simulink model "Regulation_task_cartesian_and_posture"  (R2025b)
settings: Solver=VariableStepAuto  StartTime=0.0  StopTime=10.0  RelTol=1e-3
values from neighbouring files (symbols this model uses):
  k1 = 2 * zeta * g    (= 9.6)    [test1.m]
  k2 = g^2    (= 64)    [test1.m]
  k3 = k1    (= 9.6)    [test1.m]
undefined symbols (not defined in the file or in its folder): shift_time
settings Model: Creator=david  LastModifiedBy=david

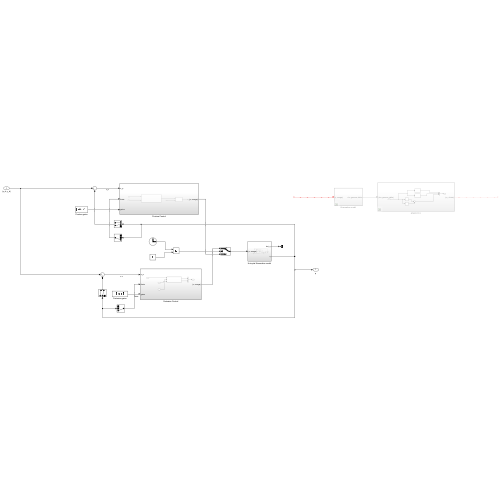
[thumbnail: Simulink's stored preview of the top-level diagram]
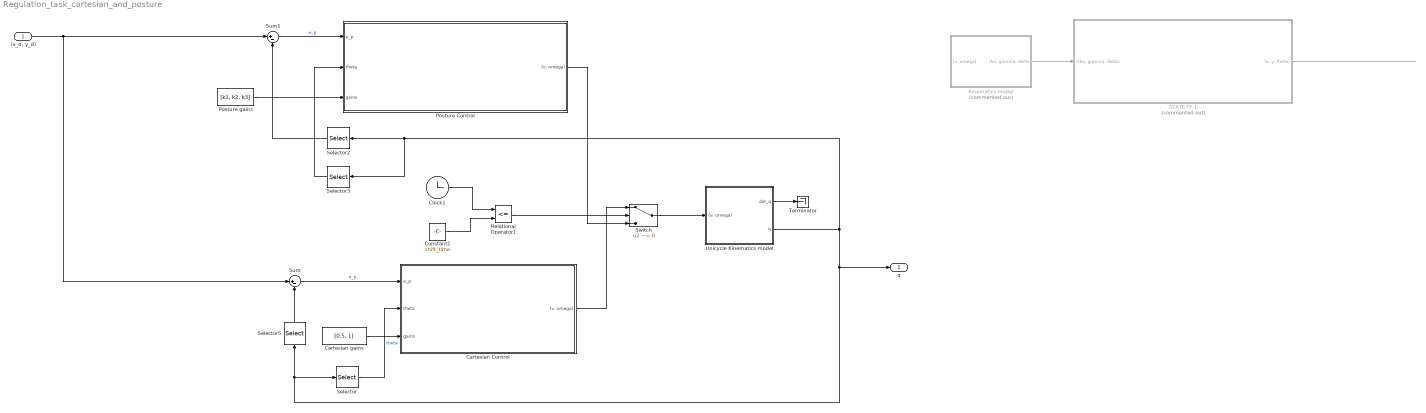
== system Regulation_task_cartesian_and_posture ==
  "(x_d, y_d)" : Inport
  Cartesian Control : Subsystem
  Cartesian gains : Constant  Value=[0.5, 1]
  Clock1 : Clock
  Constant1 : Constant  Value=shift_time
  Kinematics model : Subsystem  Commented=on
  Posture Control : Subsystem
  Posture gains : Constant  Value=[k1, k2, k3]
  Relational Operator1 : RelationalOperator  Operator=<=  OutDataTypeStr=boolean  RndMeth=Simplest  InputSameDT=off
  STATE TF-1 : Subsystem  Commented=on
  Selector : Selector  InputPortWidth=3  IndexOptions=Index vector (dialog)  Indices=[3]  OutputSizes=1
  Selector2 : Selector  InputPortWidth=3  IndexOptions=Index vector (dialog)  Indices=[1 2]  OutputSizes=1
  Selector3 : Selector  InputPortWidth=3  IndexOptions=Index vector (dialog)  Indices=[3]  OutputSizes=1
  Selector5 : Selector  InputPortWidth=3  IndexOptions=Index vector (dialog)  Indices=[1 2]  OutputSizes=1
  Sum : Sum  Inputs=|+-
  Sum1 : Sum  Inputs=|+-
  Switch : Switch  Criteria=u2 ~= 0  Threshold=0.1  SaturateOnIntegerOverflow=off  InputSameDT=off
  Terminator : Terminator
  Unicycle Kinematics model : Subsystem
  q : Outport
  wires:
  Sum/1 -> Cartesian Control/1(e_p)  "e_p"
  Selector/1 -> Cartesian Control/2(theta)  "theta"
  Unicycle Kinematics model/2(q) -> Selector3/1, Selector2/1, q/1, Selector5/1, Selector/1
  Cartesian gains/1 -> Cartesian Control/3(gains)
  STATE TF-1/1("(x, y, theta)") -> ?
  Kinematics model/1("rho, gamma, delta") -> STATE TF-1/1("(rho, gamma, delta)")
  Selector2/1 -> Sum1/2
  Sum1/1 -> Posture Control/1(e_p)  "e_p"
  Selector3/1 -> Posture Control/2(theta)
  Unicycle Kinematics model/1(dot_q) -> Terminator/1
  Cartesian Control/1("(v, omega)") -> Switch/1
  ? -> Kinematics model/1("(v, omega)")
  Switch/1 -> Unicycle Kinematics model/1("(v, omega)")
  Posture Control/1("(v, omega)") -> Switch/3
  "(x_d, y_d)"/1 -> Sum/1, Sum1/1
  Selector5/1 -> Sum/2
  Posture gains/1 -> Posture Control/3(gains)
  Relational Operator1/1 -> Switch/2
  Clock1/1 -> Relational Operator1/1
  Constant1/1 -> Relational Operator1/2

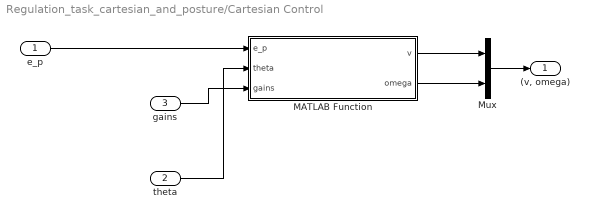
== system Regulation_task_cartesian_and_posture/Cartesian Control ==
  e_p : Inport
  theta : Inport  Port=2
  gains : Inport  Port=3
  MATLAB Function : MATLAB Function  TreatAsAtomicUnit=on
  Mux : Mux  Inputs=2
  "(v, omega)" : Outport
  wires:
  e_p/1 -> MATLAB Function/1(e_p)
  gains/1 -> MATLAB Function/3(gains)
  theta/1 -> MATLAB Function/2(theta)
  MATLAB Function/2(omega) -> Mux/2
  MATLAB Function/1(v) -> Mux/1
  Mux/1 -> "(v, omega)"/1

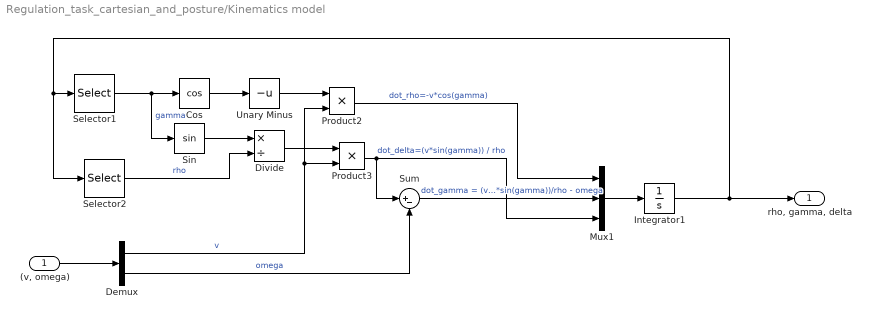
== system Regulation_task_cartesian_and_posture/Kinematics model ==
  "(v, omega)" : Inport
  Cos : Trigonometry  Operator=cos
  Demux : Demux  Outputs=2
  Divide : Product  Inputs=*/
  Integrator1 : Integrator
  Mux1 : Mux  Inputs=3
  Product2 : Product
  Product3 : Product
  Selector1 : Selector  InputPortWidth=3  IndexOptions=Index vector (dialog)  Indices=[2]  OutputSizes=1
  Selector2 : Selector  InputPortWidth=3  IndexOptions=Index vector (dialog)  Indices=[1]  OutputSizes=1
  Sin : Trigonometry
  Sum : Sum  Inputs=|+-
  Unary Minus : UnaryMinus
  "rho, gamma, delta" : Outport
  wires:
  Integrator1/1 -> "rho, gamma, delta"/1, Selector2/1, Selector1/1
  "(v, omega)"/1 -> Demux/1
  Mux1/1 -> Integrator1/1
  Selector1/1 -> Sin/1, Cos/1  "gamma"
  Cos/1 -> Unary Minus/1
  Unary Minus/1 -> Product2/1
  Demux/1 -> Product3/2, Product2/2  "v"
  Sin/1 -> Divide/1
  Selector2/1 -> Divide/2  "rho"
  Divide/1 -> Product3/1
  Product2/1 -> Mux1/1  "dot_rho=-v*cos(gamma)"
  Product3/1 -> Sum/1, Mux1/3  "dot_delta=(v*sin(gamma)) / rho"
  Sum/1 -> Mux1/2  "dot_gamma = (v*sin(gamma))/rho - omega"
  Demux/2 -> Sum/2  "omega"

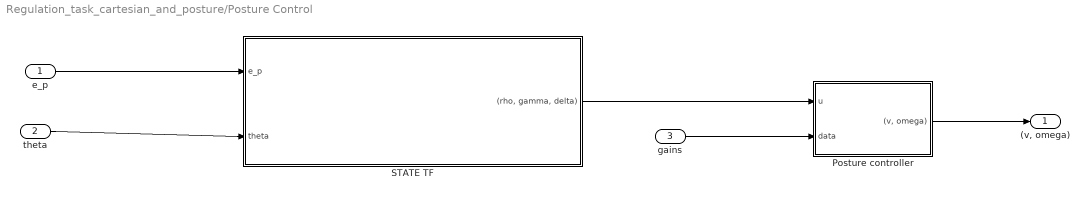
== system Regulation_task_cartesian_and_posture/Posture Control ==
  e_p : Inport
  theta : Inport  Port=2
  gains : Inport  Port=3
  Posture controller : Subsystem
  "STATE TF " : Subsystem
  "(v, omega)" : Outport
  wires:
  gains/1 -> Posture controller/2(data)
  theta/1 -> "STATE TF "/2(theta)
  "STATE TF "/1("(rho, gamma, delta)") -> Posture controller/1(u)
  Posture controller/1("(v, omega)") -> "(v, omega)"/1
  e_p/1 -> "STATE TF "/1(e_p)

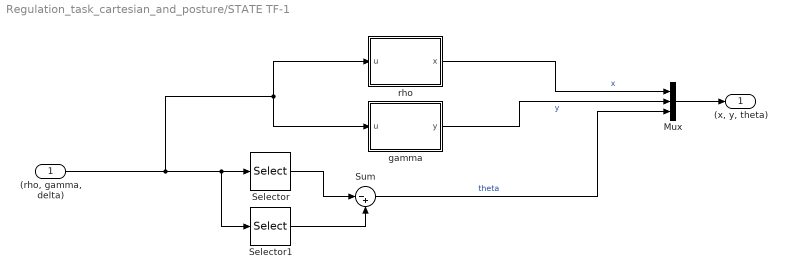
== system Regulation_task_cartesian_and_posture/STATE TF-1 ==
  "(rho, gamma, delta)" : Inport
  Mux : Mux  Inputs=3
  Selector : Selector  InputPortWidth=3  IndexOptions=Index vector (dialog)  Indices=[2]  OutputSizes=1
  Selector1 : Selector  InputPortWidth=3  IndexOptions=Index vector (dialog)  Indices=[3]  OutputSizes=1
  Sum : Sum  Inputs=|-+
  gamma : MATLAB Function  TreatAsAtomicUnit=on
  rho : MATLAB Function  TreatAsAtomicUnit=on
  "(x, y, theta)" : Outport
  wires:
  Mux/1 -> "(x, y, theta)"/1
  "(rho, gamma, delta)"/1 -> gamma/1(u), rho/1(u), Selector1/1, Selector/1
  Selector1/1 -> Sum/2
  Selector/1 -> Sum/1
  Sum/1 -> Mux/3  "theta"
  gamma/1(y) -> Mux/2  "y"
  rho/1(x) -> Mux/1  "x"

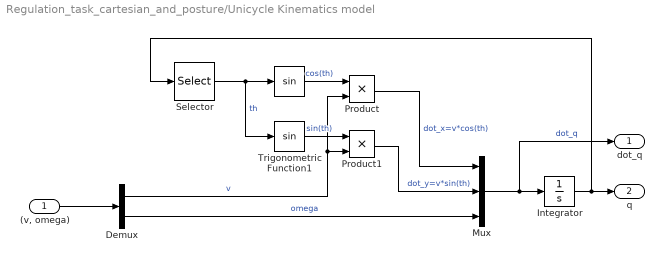
== system Regulation_task_cartesian_and_posture/Unicycle Kinematics model ==
  "(v, omega)" : Inport
  " " : Trigonometry
  Demux : Demux  Outputs=2
  Integrator : Integrator
  Mux : Mux  Inputs=3
  Product : Product
  Product1 : Product
  Selector : Selector  InputPortWidth=3  IndexOptions=Index vector (dialog)  Indices=[3]  OutputSizes=1
  Trigonometric Function1 : Trigonometry
  dot_q : Outport
  q : Outport  Port=2
  wires:
  Integrator/1 -> Selector/1, q/1
  "(v, omega)"/1 -> Demux/1
  Mux/1 -> dot_q/1, Integrator/1  "dot_q"
  Demux/2 -> Mux/3  "omega"
  Selector/1 -> Trigonometric Function1/1, " "/1  "th"
  " "/1 -> Product/1  "cos(th)"
  Trigonometric Function1/1 -> Product1/1  "sin(th)"
  Demux/1 -> Product1/2, Product/2  "v"
  Product1/1 -> Mux/2  "dot_y=v*sin(th)"
  Product/1 -> Mux/1  "dot_x=v*cos(th)"

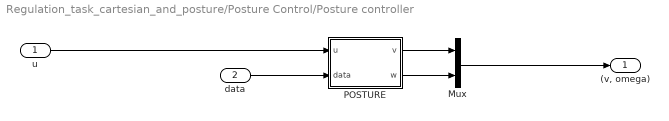
== system Regulation_task_cartesian_and_posture/Posture Control/Posture controller ==
  u : Inport
  data : Inport  Port=2
  Mux : Mux  Inputs=2
  POSTURE : MATLAB Function  TreatAsAtomicUnit=on
  "(v, omega)" : Outport
  wires:
  POSTURE/2(w) -> Mux/2
  u/1 -> POSTURE/1(u)
  Mux/1 -> "(v, omega)"/1
  data/1 -> POSTURE/2(data)
  POSTURE/1(v) -> Mux/1

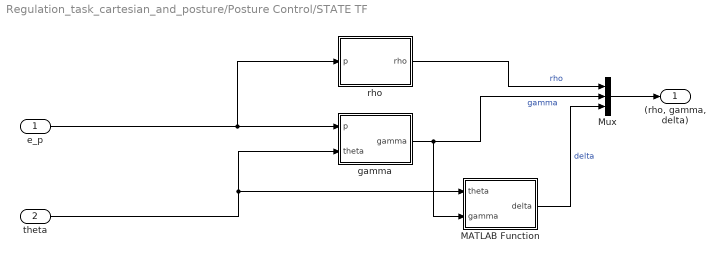
== system Regulation_task_cartesian_and_posture/Posture Control/STATE TF  ==
  e_p : Inport
  theta : Inport  Port=2
  MATLAB Function : MATLAB Function  TreatAsAtomicUnit=on
  Mux : Mux  Inputs=3
  gamma : MATLAB Function  TreatAsAtomicUnit=on
  rho : MATLAB Function  TreatAsAtomicUnit=on
  "(rho, gamma, delta)" : Outport
  wires:
  gamma/1(gamma) -> Mux/2, MATLAB Function/2(gamma)  "gamma"
  rho/1(rho) -> Mux/1  "rho"
  MATLAB Function/1(delta) -> Mux/3  "delta"
  Mux/1 -> "(rho, gamma, delta)"/1
  e_p/1 -> rho/1(p), gamma/1(p)
  theta/1 -> MATLAB Function/1(theta), gamma/2(theta)

== matlab function Regulation_task_cartesian_and_posture/Posture Control/STATE TF /MATLAB Function ==
  data: theta input; delta output; gamma input
function delta = fcn(theta, gamma)



delta = theta + gamma;
end

== matlab function Regulation_task_cartesian_and_posture/Posture Control/STATE TF /gamma ==
  data: p input; gamma output; theta input
function gamma = fcn(p, theta)

e_x = -p(1);
e_y = -p(2);

gamma = atan2(e_y,e_x) + pi - theta;

end

== matlab function Regulation_task_cartesian_and_posture/STATE TF-1/gamma ==
  data: u input; y output
function y = fcn(u)

rho = u(1);
delta = u(3);

y = - rho * sin(delta);

== matlab function Regulation_task_cartesian_and_posture/Posture Control/Posture controller/POSTURE ==
  data: v output; u input; w output; data input
function [v,w]= fcn(u, data)

K1 = data(1);
K2 = data(2);
K3 = data(3);

rho = u(1);
gamma = u(2);
delta = u(3);

v = K1 * rho * cos(gamma);

if abs(gamma) < 1e-6
    s = 1;                 % sin(gamma)/gamma -> 1
else
    s = sin(gamma)/gamma;
end
w = K2*gamma + K1*(s*cos(gamma))*(gamma + K3*delta);

== matlab function Regulation_task_cartesian_and_posture/STATE TF-1/rho ==
  data: x output; u input
function x = fcn(u)

rho = u(1);
delta = u(3);

x = - rho * cos(delta);

== matlab function Regulation_task_cartesian_and_posture/Cartesian Control/MATLAB Function ==
  data: e_p input; theta input; v output; gains input; omega output
function [v, omega] = cartesian_control(e_p, theta, gains)

x_e = e_p(1);
y_e = e_p(2);

kv = gains(1);
kw = gains(2);

% CARTESIAN_CONTROL
% Obiettivo: Portare il robot all'origine (0,0) ignorando l'orientamento finale.
    
% gamma è l'angolo tra il vettore errore e l'asse sagittale del robot.
% Formula: gamma = atan2(y, x) + pi - theta   
gamma = atan2(y_e, x_e) + pi - theta;
    
% IMPORTANTE: Normalizzazione dell'angolo
% Dobbiamo assicurarci che gamma sia tra -pi e pi, altrimenti
% il robot potrebbe fare giri su se stesso inutilmente.
gamma = atan2(sin(gamma), cos(gamma));
    
% --- 2. Calcolo Velocità Lineare v (1.216) ---
% v = kv * <ep, n> = kv * (-x*cos(theta) - y*sin(theta))
% Questa formula proietta la distanza sull'asse di avanzamento del robot.
v = kv * (x_e * cos(theta) + y_e * sin(theta));
    
% --- 3. Calcolo Velocità Angolare omega (1.217) ---
% omega = kw * gamma
% Il robot sterza per annullare l'errore angolare e puntare verso l'origine.
omega = kw * gamma;

== matlab function Regulation_task_cartesian_and_posture/Posture Control/STATE TF /rho ==
  data: rho output; p input
function rho = fcn(p)
e_x = -p(1);
e_y = -p(2);
rho = sqrt(e_x^2 + e_y^2);
end
